simulink model "ObjectTrackingMove"  (R2019a)
settings: Solver=FixedStepAuto  StartTime=0.0  StopTime=inf  RelTol=1e-3  EnableMultiTasking=on
undefined symbols (not defined in the file or in its folder): DiscIntNeverNeededParam
libraries: embdlinuxlib x24, raspberrypilib x2, dspswit3 x1, simulink x1
settings Model: SimulationMode=external  Creator=wojna  LastModifiedBy=asia1
settings SolverCC: PositivePriorityOrder=on
settings OptimizationCC: EnhancedBackFolding=on  PassReuseOutputArgsAs=Individual arguments  MaxStackSize=64  OptimizeBlockOrder=speed  DifferentSizesBufferReuse=on  OptimizationCustomize=off
settings DebuggingCC: ParameterTunabilityLossMsg=error
settings HardwareCC: ProdBitPerPointer=32  ProdBitPerSizeT=32  ProdBitPerPtrDiffT=32  ProdLargestAtomicInteger=Long  ProdLargestAtomicFloat=Double  ProdWordSize=32  ProdLongLongMode=on  ProdHWDeviceType=ARM Compatible->ARM Cortex  UseEmbeddedCoderFeatures=off  UseSimulinkCoderFeatures=off
settings SFSimCC: MATLABDynamicMemAlloc=off
settings RTWCC: SystemTargetFile=ert.tlc  HardwareBoard=Raspberry Pi  TLCOptions="-aInlineSetEventsForThisBaseRateFcn=TLC_FALSE -aSuppressMultiTaskScheduler=TLC_FALSE  -aRateBasedStepFcn=0"  TemplateMakefile=ert_default_tmf  GenerateReport=on  Toolchain=GNU GCC Raspberry Pi  BuildConfiguration=Faster Runs  IncludeHyperlinkInReport=on  LaunchReport=on  GenerateTraceInfo=on  GenerateTraceReport=on  GenerateTraceReportSl=on  GenerateTraceReportSf=on  GenerateTraceReportEml=on
settings CodeAppCC: ForceParamTrailComments=on  IgnoreCustomStorageClasses=off  OperatorAnnotations=on  SimulinkDataObjDesc=on  SFDataObjDesc=on  MangleLength=10  InsertBlockDesc=on
settings ERTTargetCC: SupportNonInlinedSFcns=on  SupportVariableSizeSignals=on

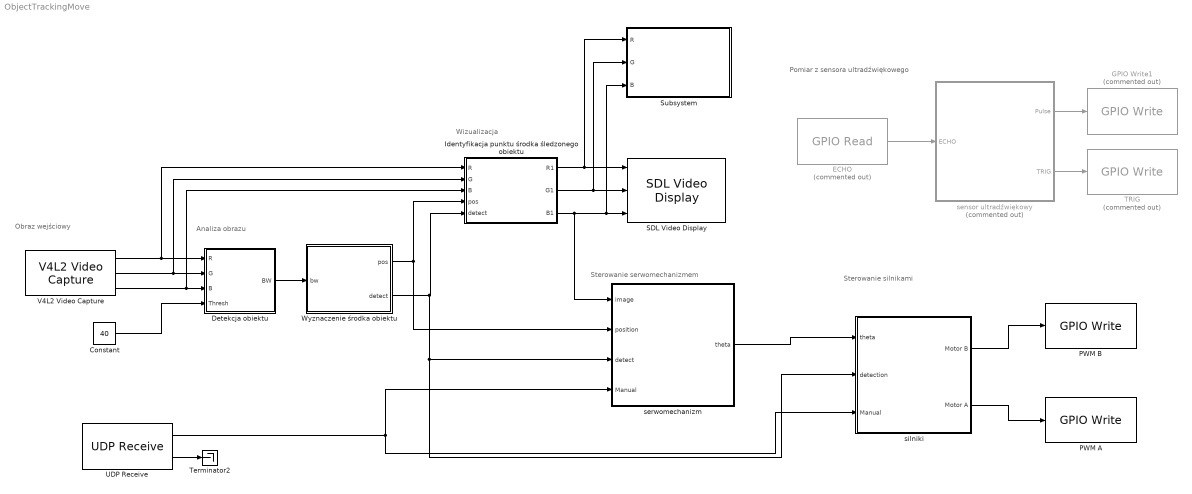
== system ObjectTrackingMove ==
  note: Obraz wejściowy
  note: Pomiar z sensora ultradźwiękowego
  note: Wizualizacja
  note: Analiza obrazu
  note: Sterowanie serwomechanizmem
  note: Sterowanie silnikami
  Constant : Constant  Value=40
  Detekcja obiektu : Subsystem
  ECHO : embdlinuxlib/GPIO Read  Commented=on  board=Pi 3 Model B+  gpio=23  internalResistor=Off  sampleTime=2.5e-05  direction=Input  blockPlatform=Raspberry Pi
      settings: SourceProductName=Simulink Coder Support Package for BeagleBone Blue Hardware  SourceProductBaseCode=SC_BEAGLEBONE_BLUE
  GPIO Write1 : embdlinuxlib/GPIO Write  Commented=on  board=Pi 3 Model B+  gpio=24  direction=Output  blockPlatform=Raspberry Pi
      settings: SourceProductName=Simulink Coder Support Package for BeagleBone Blue Hardware  SourceProductBaseCode=SC_BEAGLEBONE_BLUE
  Identyfikacja punktu środka śledzonego obiektu : MATLAB Function  TreatAsAtomicUnit=on
  PWM A : embdlinuxlib/GPIO Write  board=Pi 3 Model B+  gpio=16  direction=Output  blockPlatform=Raspberry Pi
      settings: SourceProductName=Simulink Coder Support Package for BeagleBone Blue Hardware  SourceProductBaseCode=SC_BEAGLEBONE_BLUE
  PWM B : embdlinuxlib/GPIO Write  board=Pi 3 Model B+  gpio=20  direction=Output  blockPlatform=Raspberry Pi
      settings: SourceProductName=Simulink Coder Support Package for BeagleBone Blue Hardware  SourceProductBaseCode=SC_BEAGLEBONE_BLUE
  SDL Video Display : embdlinuxlib/SDL Video Display  pixelFormat=RGB  pixelOrder=Planar  rowMajor=on  blockPlatform=Raspberry Pi
      settings: SourceProductName=Simulink Coder Support Package for BeagleBone Blue Hardware  SourceProductBaseCode=SC_BEAGLEBONE_BLUE
  Subsystem : Subsystem
  TRIG : embdlinuxlib/GPIO Write  Commented=on  board=Pi 3 Model B+  gpio=4  direction=Output  blockPlatform=Raspberry Pi
      settings: SourceProductName=Simulink Coder Support Package for BeagleBone Blue Hardware  SourceProductBaseCode=SC_BEAGLEBONE_BLUE
  Terminator2 : Terminator
  UDP Receive : embdlinuxlib/UDP Receive  localURL='0.0.0.0'  localPort=26000  remoteURL='0.0.0.0'  remotePort=-1  recvBufferSize=8192  signalDatatype=single  dims=1  isVarSize=off  showBlockingTime=off  blockingTime=0  sampletime=0.01  blockPlatform=Raspberry Pi
      settings: SourceProductName=Simulink Coder Support Package for BeagleBone Blue Hardware  SourceProductBaseCode=SC_BEAGLEBONE_BLUE
  V4L2 Video Capture : embdlinuxlib/V4L2 Video Capture  m_devName='/dev/video0'  roi=[0, 0, 640, 480]  imSizeSelection=160x120  imSize=[640, 480]  pixelFormat=RGB  pixelOrder=Planar  sampleTime=0.01  simOutput=Colorbars  blockPlatform=Raspberry Pi
      settings: SourceProductName=Simulink Coder Support Package for BeagleBone Blue Hardware  SourceProductBaseCode=SC_BEAGLEBONE_BLUE
  Wyznaczenie środka obiektu : MATLAB Function  TreatAsAtomicUnit=on
  sensor ultradźwiękowy : Subsystem  Commented=on
  serwomechanizm : Subsystem
  silniki : Subsystem
  wires:
  V4L2 Video Capture/1 -> Detekcja obiektu/1(R), Identyfikacja punktu środka śledzonego obiektu/1(R)
  V4L2 Video Capture/2 -> Detekcja obiektu/2(G), Identyfikacja punktu środka śledzonego obiektu/2(G)
  V4L2 Video Capture/3 -> Identyfikacja punktu środka śledzonego obiektu/3(B), Detekcja obiektu/3(B)
  Detekcja obiektu/1(BW) -> Wyznaczenie środka obiektu/1(bw)
  Wyznaczenie środka obiektu/1(pos) -> Identyfikacja punktu środka śledzonego obiektu/4(pos), serwomechanizm/2(position)
  Wyznaczenie środka obiektu/2(detect) -> serwomechanizm/3(detect), silniki/2(detection), Identyfikacja punktu środka śledzonego obiektu/5(detect)
  Identyfikacja punktu środka śledzonego obiektu/1(R1) -> Subsystem/1("R "), SDL Video Display/1
  Identyfikacja punktu środka śledzonego obiektu/2(G1) -> Subsystem/2("G "), SDL Video Display/2
  Identyfikacja punktu środka śledzonego obiektu/3(B1) -> serwomechanizm/1(image), Subsystem/3(B), SDL Video Display/3
  Constant/1 -> Detekcja obiektu/4(Thresh)
  serwomechanizm/1(theta) -> silniki/1(theta)
  sensor ultradźwiękowy/2(TRIG) -> TRIG/1
  ECHO/1 -> sensor ultradźwiękowy/1(ECHO)
  sensor ultradźwiękowy/1(Pulse) -> GPIO Write1/1
  silniki/2(Motor A) -> PWM A/1
  silniki/1(Motor B) -> PWM B/1
  UDP Receive/2 -> Terminator2/1
  UDP Receive/1 -> silniki/3(Manual), serwomechanizm/4(Manual)

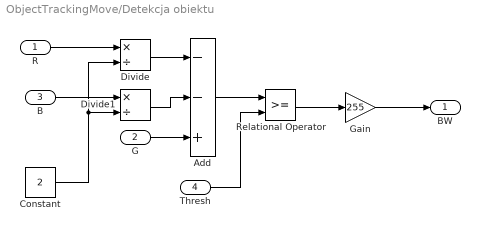
== system ObjectTrackingMove/Detekcja obiektu ==
  R : Inport
  G : Inport  Port=2
  B : Inport  Port=3
  Thresh : Inport  Port=4
  Add : Sum  Inputs=--+
  Constant : Constant  Value=2
  Divide : Product  Inputs=*/
  Divide1 : Product  Inputs=*/
  Gain : Gain  Gain=255
  Relational Operator : RelationalOperator  OutDataTypeStr=boolean  RndMeth=Simplest
  BW : Outport
  wires:
  Thresh/1 -> Relational Operator/2
  Constant/1 -> Divide1/2, Divide/2
  Gain/1 -> BW/1
  Add/1 -> Relational Operator/1
  Divide1/1 -> Add/2
  Relational Operator/1 -> Gain/1
  Divide/1 -> Add/1
  R/1 -> Divide/1
  B/1 -> Divide1/1
  G/1 -> Add/3

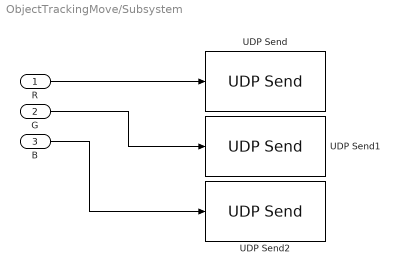
== system ObjectTrackingMove/Subsystem ==
  "R " : Inport
  "G " : Inport  Port=2
  B : Inport  Port=3
  UDP Send : embdlinuxlib/UDP Send  remoteURL='192.168.0.100'  remotePort=26010  localURL='255.255.255.255'  localPortSource=Automatically determine  localPort=-1  sampletime=-1  blockPlatform=Raspberry Pi  separateLengthPort=0
      settings: SourceProductName=Simulink Coder Support Package for BeagleBone Blue Hardware  SourceProductBaseCode=SC_BEAGLEBONE_BLUE
  UDP Send1 : embdlinuxlib/UDP Send  remoteURL='192.168.0.100'  remotePort=26011  localURL='255.255.255.255'  localPortSource=Automatically determine  localPort=-1  sampletime=-1  blockPlatform=Raspberry Pi  separateLengthPort=0
      settings: SourceProductName=Simulink Coder Support Package for BeagleBone Blue Hardware  SourceProductBaseCode=SC_BEAGLEBONE_BLUE
  UDP Send2 : embdlinuxlib/UDP Send  remoteURL='192.168.0.100'  remotePort=26012  localURL='255.255.255.255'  localPortSource=Automatically determine  localPort=-1  sampletime=-1  blockPlatform=Raspberry Pi  separateLengthPort=0
      settings: SourceProductName=Simulink Coder Support Package for BeagleBone Blue Hardware  SourceProductBaseCode=SC_BEAGLEBONE_BLUE
  wires:
  "R "/1 -> UDP Send/1
  "G "/1 -> UDP Send1/1
  B/1 -> UDP Send2/1

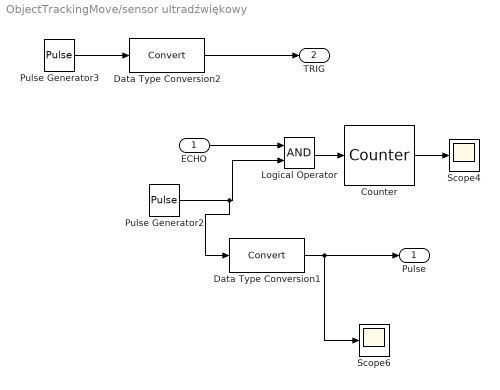
== system ObjectTrackingMove/sensor ultradźwiękowy ==
  ECHO : Inport
  Counter : dspswit3/Counter  Direction=Up  CountEvent=Rising edge  CounterSize=8 bits  MaxCount=255  InitialCount=0  Output=Count  HitValue=32  ResetInput=off  SamplesPerFrame=1  Ts=1  CntDtype=double  HitDtype=Logical
  Data Type Conversion1 : DataTypeConversion
  Data Type Conversion2 : DataTypeConversion
  Logical Operator : Logic  AllPortsSameDT=off  OutDataTypeStr=boolean
  Pulse Generator2 : DiscretePulseGenerator  PulseType=Time based  Amplitude=3  Period=0.00005  PulseWidth=50
  Pulse Generator3 : DiscretePulseGenerator  PulseType=Time based  Amplitude=3  Period=0.1  PulseWidth=0.01
  Scope4 : Scope
  Scope6 : Scope
  Pulse : Outport
  TRIG : Outport  Port=2
  wires:
  Data Type Conversion1/1 -> Pulse/1, Scope6/1
  Counter/1 -> Scope4/1
  Pulse Generator3/1 -> Data Type Conversion2/1
  Pulse Generator2/1 -> Logical Operator/2, Data Type Conversion1/1
  ECHO/1 -> Logical Operator/1
  Logical Operator/1 -> Counter/1
  Data Type Conversion2/1 -> TRIG/1

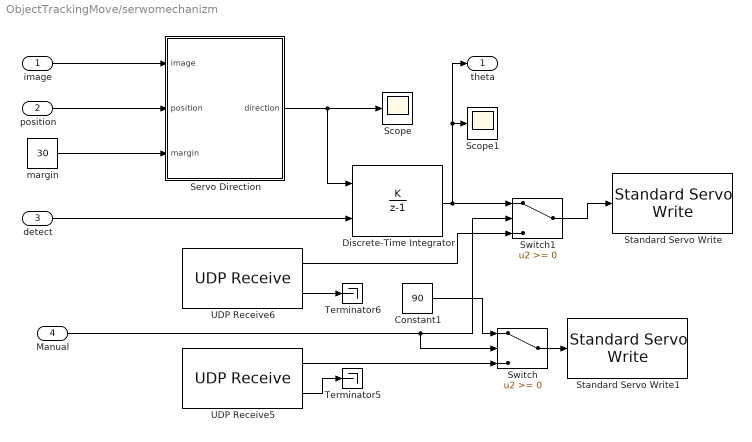
== system ObjectTrackingMove/serwomechanizm ==
  image : Inport
  position : Inport  Port=2
  detect : Inport  Port=3
  Manual : Inport  Port=4
  Constant1 : Constant  Value=90
  Discrete-Time Integrator : DiscreteIntegrator  IntegratorMethod=Accumulation: Forward Euler  ExternalReset=falling  InitialCondition=90  SampleTime=-1  LimitOutput=on  UpperSaturationLimit=180  LowerSaturationLimit=0  ICPrevOutput=DiscIntNeverNeededParam  ICPrevScaledInput=DiscIntNeverNeededParam
  Scope : Scope
  Scope1 : Scope
  "Servo Direction " : Subsystem
  Standard Servo Write : raspberrypilib/Standard Servo Write  board=Pi 3 Model B  Pin_=26  MinPulseDuration=1000e-6  MaxPulseDuration=2000e-6  blockPlatform=Raspberry Pi
      settings: SourceProductName=Simulink Support Package for Raspberry Pi Hardware  SourceProductBaseCode=RASPPI
  Standard Servo Write1 : raspberrypilib/Standard Servo Write  board=Pi 3 Model B  Pin_=19  MinPulseDuration=1000e-6  MaxPulseDuration=2000e-6  blockPlatform=Raspberry Pi
      settings: SourceProductName=Simulink Support Package for Raspberry Pi Hardware  SourceProductBaseCode=RASPPI
  Switch : Switch
  Switch1 : Switch
  Terminator5 : Terminator
  Terminator6 : Terminator
  UDP Receive5 : embdlinuxlib/UDP Receive  localURL='0.0.0.0'  localPort=26001  remoteURL='0.0.0.0'  remotePort=-1  recvBufferSize=8192  signalDatatype=single  dims=1  isVarSize=off  showBlockingTime=off  blockingTime=0  sampletime=0.01  blockPlatform=Raspberry Pi
      settings: SourceProductName=Simulink Coder Support Package for BeagleBone Blue Hardware  SourceProductBaseCode=SC_BEAGLEBONE_BLUE
  UDP Receive6 : embdlinuxlib/UDP Receive  localURL='0.0.0.0'  localPort=26002  remoteURL='0.0.0.0'  remotePort=-1  recvBufferSize=8192  signalDatatype=single  dims=1  isVarSize=off  showBlockingTime=off  blockingTime=0  sampletime=0.01  blockPlatform=Raspberry Pi
      settings: SourceProductName=Simulink Coder Support Package for BeagleBone Blue Hardware  SourceProductBaseCode=SC_BEAGLEBONE_BLUE
  margin : Constant  Value=30
  theta : Outport
  wires:
  "Servo Direction "/1("direction ") -> Discrete-Time Integrator/1, Scope/1
  detect/1 -> Discrete-Time Integrator/2
  Discrete-Time Integrator/1 -> theta/1, Scope1/1, Switch1/1
  margin/1 -> "Servo Direction "/3("margin ")
  position/1 -> "Servo Direction "/2(position)
  image/1 -> "Servo Direction "/1(image)
  UDP Receive5/2 -> Terminator5/1
  UDP Receive6/2 -> Terminator6/1
  UDP Receive6/1 -> Switch1/3
  Switch/1 -> Standard Servo Write1/1
  Constant1/1 -> Switch/1
  UDP Receive5/1 -> Switch/3
  Manual/1 -> Switch1/2, Switch/2
  Switch1/1 -> Standard Servo Write/1

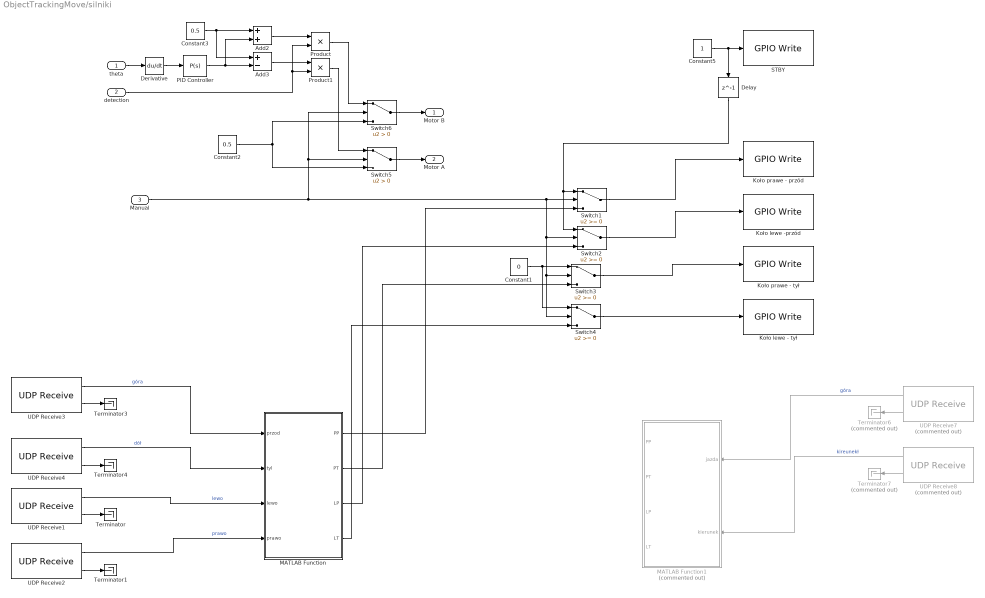
== system ObjectTrackingMove/silniki ==
  theta : Inport
  detection : Inport  Port=2
  Manual : Inport  Port=3
  Add2 : Sum
  Add3 : Sum  Inputs=+-
  Constant1 : Constant  Value=0
  Constant2 : Constant  Value=0.5
  Constant3 : Constant  Value=0.5
  Constant5 : Constant
  Delay : Delay  DelayLength=1  InitialCondition=0
  Derivative : Derivative
  Koło lewe - tył : embdlinuxlib/GPIO Write  board=Pi 3 Model B+  gpio=17  direction=Output  blockPlatform=Raspberry Pi
      settings: SourceProductName=Simulink Coder Support Package for BeagleBone Blue Hardware  SourceProductBaseCode=SC_BEAGLEBONE_BLUE
  Koło lewe -przód : embdlinuxlib/GPIO Write  board=Pi 3 Model B+  gpio=18  direction=Output  blockPlatform=Raspberry Pi
      settings: SourceProductName=Simulink Coder Support Package for BeagleBone Blue Hardware  SourceProductBaseCode=SC_BEAGLEBONE_BLUE
  Koło prawe - przód : embdlinuxlib/GPIO Write  board=Pi 3 Model B+  gpio=22  direction=Output  blockPlatform=Raspberry Pi
      settings: SourceProductName=Simulink Coder Support Package for BeagleBone Blue Hardware  SourceProductBaseCode=SC_BEAGLEBONE_BLUE
  Koło prawe - tył : embdlinuxlib/GPIO Write  board=Pi 3 Model B+  gpio=27  direction=Output  blockPlatform=Raspberry Pi
      settings: SourceProductName=Simulink Coder Support Package for BeagleBone Blue Hardware  SourceProductBaseCode=SC_BEAGLEBONE_BLUE
  MATLAB Function : MATLAB Function  TreatAsAtomicUnit=on
  MATLAB Function1 : MATLAB Function  Commented=on  TreatAsAtomicUnit=on
  PID Controller : simulink/Continuous/PID Controller  Controller=P  Form=Parallel  TimeDomain=Continuous-time  SampleTime=-1  IntegratorMethod=Forward Euler  FilterMethod=Forward Euler  ControllerParametersSource=internal  P=1.5  I=1  D=0  UseFilter=on  N=100  TunerSelectOption=Transfer Function Based (PID Tuner App)  InitialConditionSource=internal  InitialConditionForIntegrator=0  InitialConditionForFilter=0  DifferentiatorICPrevScaledInput=0  ExternalReset=none  TrackingMode=off  Kt=1  LimitOutput=off  UpperSaturationLimit=inf  LowerSaturationLimit=-inf  LinearizeAsGain=on  AntiWindupMode=none  Kb=1  POutMin=[]  POutMax=[]  IOutMin=[]  IOutMax=[]  DOutMin=[]  DOutMax=[]  NOutMin=[]  NOutMax=[]  SumOutMin=[]  SumOutMax=[]  SaturationOutMin=[]  SaturationOutMax=[]  PParamMin=[]  PParamMax=[]  IParamMin=[]  IParamMax=[]  DParamMin=[]  DParamMax=[]  NParamMin=[]  NParamMax=[]  KbParamMin=[]  KbParamMax=[]  KtParamMin=[]  KtParamMax=[]  KbOutMin=[]  KbOutMax=[]  KtOutMin=[]  KtOutMax=[]  IntegratorOutMin=[]  IntegratorOutMax=[]  FilterOutMin=[]  FilterOutMax=[]  SumI1OutMin=[]  SumI1OutMax=[]  SumI2OutMin=[]  SumI2OutMax=[]  SumI3OutMin=[]  SumI3OutMax=[]  SumI4OutMin=[]  SumI4OutMax=[]  SumDOutMin=[]  SumDOutMax=[]  DifferentiatorOutMin=[]  DifferentiatorOutMax=[]  FilterDiffOutCoefMin=[]  FilterDiffOutCoefMax=[]  ReciprocalOutMin=[]  ReciprocalOutMax=[]  SumDenOutMin=[]  SumDenOutMax=[]  SumNumOutMin=[]  SumNumOutMax=[]  DivideOutMin=[]  DivideOutMax=[]  IntegratorContinuousStateAttributes=''  IntegratorStateMustResolveToSignalObject=off  IntegratorRTWStateStorageClass=Auto  FilterContinuousStateAttributes=''  FilterStateMustResolveToSignalObject=off  FilterRTWStateStorageClass=Auto  ParallelPVariant=InternalParameters  IdealPVariant=Disabled  IVariant=Disabled  DVariant=Disabled  IntegratorVariant=Disabled  SatVariant=Disabled  AWVariant=Disabled  PCopyVariant=Disabled  TRVariant=Disabled  FdbkBlocksVariant=Forward  IdealPFdbkVariant=Disabled  SatFdbkVariant=Disabled  DerivativeFilterVariant=Disabled  NVariant=Disabled  NCopyVariant=Disabled_SignalSpec  FilterICVariant=Disabled  IntegratorICVariant=Disabled  ExternalResetVariant=Disabled  TRSumVariant=Passthrough  SumFdbkVariant=Disabled  SumVariant=Passthrough_P
  Product : Product
  Product1 : Product
  STBY : embdlinuxlib/GPIO Write  board=Pi 3 Model B+  gpio=21  direction=Output  blockPlatform=Raspberry Pi
      settings: SourceProductName=Simulink Coder Support Package for BeagleBone Blue Hardware  SourceProductBaseCode=SC_BEAGLEBONE_BLUE
  Switch{1..4} (4 alike) : Switch
  Switch5 : Switch  Criteria=u2 > Threshold
  Switch6 : Switch  Criteria=u2 > Threshold
  Terminator{,1,3..4} (4 alike) : Terminator
  Terminator6 : Terminator  Commented=on
  Terminator7 : Terminator  Commented=on
  UDP Receive1 : embdlinuxlib/UDP Receive  localURL='0.0.0.0'  localPort=26005  remoteURL='0.0.0.0'  remotePort=-1  recvBufferSize=8192  signalDatatype=single  dims=1  isVarSize=off  showBlockingTime=off  blockingTime=0  sampletime=0.01  blockPlatform=Raspberry Pi
      settings: SourceProductName=Simulink Coder Support Package for BeagleBone Blue Hardware  SourceProductBaseCode=SC_BEAGLEBONE_BLUE
  UDP Receive2 : embdlinuxlib/UDP Receive  localURL='0.0.0.0'  localPort=26006  remoteURL='0.0.0.0'  remotePort=-1  recvBufferSize=8192  signalDatatype=single  dims=1  isVarSize=off  showBlockingTime=off  blockingTime=0  sampletime=0.01  blockPlatform=Raspberry Pi
      settings: SourceProductName=Simulink Coder Support Package for BeagleBone Blue Hardware  SourceProductBaseCode=SC_BEAGLEBONE_BLUE
  UDP Receive3 : embdlinuxlib/UDP Receive  localURL='0.0.0.0'  localPort=26003  remoteURL='0.0.0.0'  remotePort=-1  recvBufferSize=8192  signalDatatype=single  dims=1  isVarSize=off  showBlockingTime=off  blockingTime=0  sampletime=0.01  blockPlatform=Raspberry Pi
      settings: SourceProductName=Simulink Coder Support Package for BeagleBone Blue Hardware  SourceProductBaseCode=SC_BEAGLEBONE_BLUE
  UDP Receive4 : embdlinuxlib/UDP Receive  localURL='0.0.0.0'  localPort=26004  remoteURL='0.0.0.0'  remotePort=-1  recvBufferSize=8192  signalDatatype=single  dims=1  isVarSize=off  showBlockingTime=off  blockingTime=0  sampletime=0.01  blockPlatform=Raspberry Pi
      settings: SourceProductName=Simulink Coder Support Package for BeagleBone Blue Hardware  SourceProductBaseCode=SC_BEAGLEBONE_BLUE
  UDP Receive7 : embdlinuxlib/UDP Receive  Commented=on  localURL='0.0.0.0'  localPort=26003  remoteURL='0.0.0.0'  remotePort=-1  recvBufferSize=8192  signalDatatype=single  dims=1  isVarSize=off  showBlockingTime=off  blockingTime=0  sampletime=0.01  blockPlatform=Raspberry Pi
      settings: SourceProductName=Simulink Coder Support Package for BeagleBone Blue Hardware  SourceProductBaseCode=SC_BEAGLEBONE_BLUE
  UDP Receive8 : embdlinuxlib/UDP Receive  Commented=on  localURL='0.0.0.0'  localPort=26004  remoteURL='0.0.0.0'  remotePort=-1  recvBufferSize=8192  signalDatatype=single  dims=1  isVarSize=off  showBlockingTime=off  blockingTime=0  sampletime=0.01  blockPlatform=Raspberry Pi
      settings: SourceProductName=Simulink Coder Support Package for BeagleBone Blue Hardware  SourceProductBaseCode=SC_BEAGLEBONE_BLUE
  Motor B : Outport
  Motor A : Outport  Port=2
  wires:
  Add2/1 -> Product/1
  Constant3/1 -> Add3/1, Add2/1
  PID Controller/1 -> Add3/2, Add2/2
  Derivative/1 -> PID Controller/1
  Add3/1 -> Product1/1
  theta/1 -> Derivative/1
  detection/1 -> Product/2, Product1/2
  Constant5/1 -> STBY/1, Delay/1
  Delay/1 -> Switch2/1, Switch1/1
  Manual/1 -> Switch6/2, Switch5/2, Switch4/2, Switch3/2, Switch2/2, Switch1/2
  UDP Receive3/2 -> Terminator3/1
  UDP Receive4/2 -> Terminator4/1
  UDP Receive1/2 -> Terminator/1
  UDP Receive1/1 -> MATLAB Function/3(lewo)  "lewo"
  UDP Receive3/1 -> MATLAB Function/1(przod)  "góra"
  UDP Receive4/1 -> MATLAB Function/2(tyl)  "dół"
  UDP Receive2/2 -> Terminator1/1
  UDP Receive2/1 -> MATLAB Function/4(prawo)  "prawo"
  Switch4/1 -> Koło lewe - tył/1
  Constant1/1 -> Switch4/1, Switch3/1
  Switch1/1 -> Koło prawe - przód/1
  Switch2/1 -> Koło lewe -przód/1
  Switch3/1 -> Koło prawe - tył/1
  Switch6/1 -> Motor B/1
  Product/1 -> Switch6/1
  Product1/1 -> Switch5/1
  Switch5/1 -> Motor A/1
  Constant2/1 -> Switch5/3, Switch6/3
  UDP Receive7/1 -> MATLAB Function1/1(jazda)  "góra"
  UDP Receive8/1 -> MATLAB Function1/2(kierunek)  "kireunekł"
  UDP Receive7/2 -> Terminator6/1
  UDP Receive8/2 -> Terminator7/1
  MATLAB Function/1(PP) -> Switch1/3
  MATLAB Function/2(PT) -> Switch3/3
  MATLAB Function/3(LP) -> Switch2/3
  MATLAB Function/4(LT) -> Switch4/3

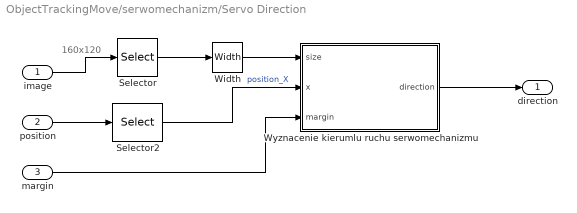
== system ObjectTrackingMove/serwomechanizm/Servo Direction  ==
  note: 160x120
  image : Inport
  position : Inport  Port=2
  "margin " : Inport  Port=3
  Selector : Selector  NumberOfDimensions=2  InputPortWidth=160  IndexOptions=Select all,Starting index (dialog)  Indices=1,1  OutputSizes=160,1
  Selector2 : Selector  InputPortWidth=2  IndexOptions=Index vector (dialog)  Indices=1  OutputSizes=1
  Width : Width
  Wyznacenie kierumlu ruchu serwomechanizmu : MATLAB Function  TreatAsAtomicUnit=on
  "direction " : Outport
  wires:
  position/1 -> Selector2/1
  Wyznacenie kierumlu ruchu serwomechanizmu/1(direction) -> "direction "/1
  Selector2/1 -> Wyznacenie kierumlu ruchu serwomechanizmu/2(x)  "position_X"
  Width/1 -> Wyznacenie kierumlu ruchu serwomechanizmu/1(size)
  Selector/1 -> Width/1
  image/1 -> Selector/1
  "margin "/1 -> Wyznacenie kierumlu ruchu serwomechanizmu/3(margin)

== matlab function ObjectTrackingMove/Wyznaczenie środka obiektu ==
  data: bw input; pos output; detect output
function [pos, detect] = FindCentroid(bw)

[r,c]=find(bw);
if isempty(r)
    pos = [-1 -1];
    detect = false;
else
    pos = [mean(r), mean(c)];
    detect = true;
end

== matlab function ObjectTrackingMove/Identyfikacja punktu środka śledzonego obiektu ==
  data: R input; R1 output; G input; B input; pos input; detect input; G1 output; B1 output
function [R1,G1,B1] = MarkImage(R,G,B, pos, detect)
R1 = R; G1 = G; B1 = B;
if detect
    R1(pos(1)-3:pos(1)+3, pos(2)-3:pos(2)+3) = 255;
    G1(pos(1)-3:pos(1)+3, pos(2)-3:pos(2)+3) = 0; 
    B1(pos(1)-3:pos(1)+3, pos(2)-3:pos(2)+3) = 0;
end

== matlab function ObjectTrackingMove/serwomechanizm/Servo Direction /Wyznacenie kierumlu ruchu serwomechanizmu ==
  data: size input; direction output; x input; margin input
function direction = servoDirection(size, x, margin)

center = size/2;
if x == -1
    direction = 0;
elseif x >= center + margin
    direction = -1;
elseif x <= center - margin
    direction = 1;
else 
    direction = 0;
end

== matlab function ObjectTrackingMove/silniki/MATLAB Function ==
  data: przod input; PP output; tyl input; lewo input; prawo input; PT output; LP output; LT output
function [PP,PT,LP,LT] = Sterowanie(przod, tyl, lewo, prawo)
PP=0;
PT=0;
LP=0;
LT=0;
if przod == 1 && tyl == 0 && lewo == 0 && prawo ==0
    PP=1;
    PT=0;
    LP=1;
    LT=0;
elseif przod == 0 && tyl == 1 && lewo == 0 && prawo ==0
    PP=0;
    PT=1;
    LP=0;
    LT=1;
elseif przod == 0 && tyl == 0 && lewo == 1 && prawo ==0
    PP=1;
    PT=0;
    LP=0;
    LT=0;
elseif przod == 0 && tyl == 0 && lewo == 0 && prawo ==1
    PP=0;
    PT=0;
    LP=1;
    LT=0;
end
        
end

== matlab function ObjectTrackingMove/silniki/MATLAB Function1 ==
  data: jazda input; PP output; kierunek input; PT output; LP output; LT output
function [PP,PT,LP,LT] = Sterowanie(jazda, kierunek)
PP=0;
PT=0;
LP=0;
LT=0;
if jazda == 2 && kierunek == 1
    PP=1;
    PT=0;
    LP=1;
    LT=0;
elseif jazda == 0 && kierunek == 1
    PP=0;
    PT=1;
    LP=0;
    LT=1;
elseif jazda == 1 && kierunek == 0
    PP=1;
    PT=0;
    LP=0;
    LT=0;
elseif jazda == 1 && kierunek == 2
    PP=0;
    PT=0;
    LP=1;
    LT=0;
else
    PP=0;
    PT=0;
    LP=0;
    LT=0;
end
        
end
